simulink model "Autopilotage"  (R2022a)
settings: Solver=VariableStepAuto  StartTime=0.0  StopTime=2  FixedStep=1e-5  MaxStep=1e-4  RelTol=1e-3
undefined symbols (not defined in the file): R0
libraries: spsIGBTDiodeLib x6, spsPWMGenerator2LevelLib x3, spsAsynchronousMachineSIUnitsLib x1, spsDCVoltageSourceLib x1, spsRMSLib x1, spsVoltageMeasurementLib x1, spspowerguiLib x1
settings Model: Creator=kholo  LastModifiedBy=Dell

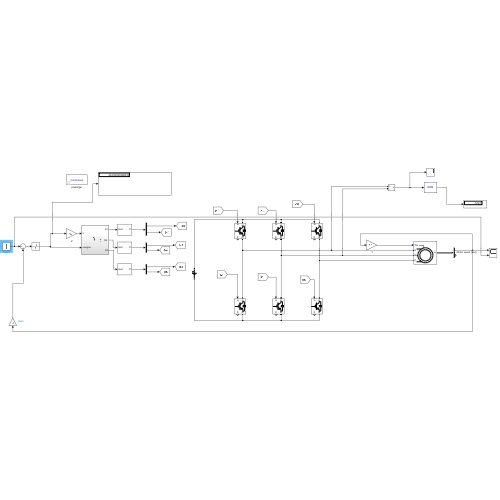
[thumbnail: Simulink's stored preview of the top-level diagram]
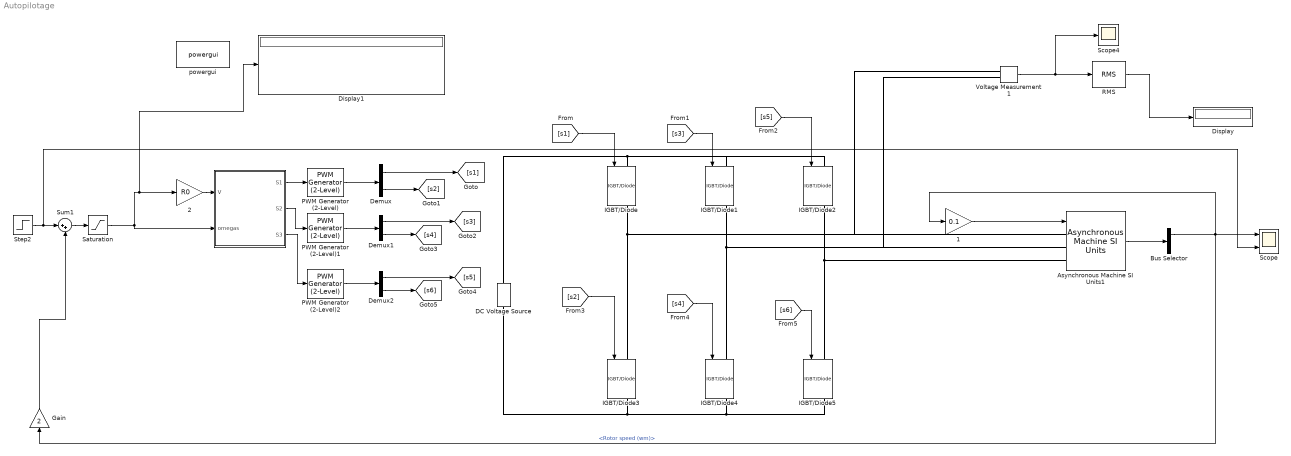
== system Autopilotage ==
  "  " : Subsystem
  " 1" : Gain  Gain=0.1
  " 2" : Gain  Gain=R0
  Asynchronous Machine SI Units1 : spsAsynchronousMachineSIUnitsLib/Asynchronous Machine SI Units  RotorType=Squirrel-cage  PresetModel=No  MechanicalLoad=Torque Tm  ShowDetailedParameters=on  ReferenceFrame=Rotor  Units=SI  MeasurementBus=off  NominalParameters=[1.845e+04 400 50]  VoltageRatio=1  Stator=[0.5968 0.0003495]  Rotor=[0.6258 0.005473]  Cage1=[0.4155 0.002066]  Cage2=[0.4168 0.0003495]  Lm=0.0354  Mechanical=[0.05 0.005879 2]  PolePairs=2  InitialConditions=[0 0 0 0 0 0 0 0]  SimulateSaturation=off  Saturation=[14.03593122, 27.81365428, 53.79336849, 72.68890987, 97.98006896, 148.6815601, 215.7428561, 302.9841135, 428.7778367 ; 230, 322, 414, 460, 506, 552, 598, 644, 690]  LoadFlowParameters=1492000  TsPowergui=0  TsBlock=-1  IterativeModel=Trapezoidal non iterative  IterativeDiscreteModel=Trapezoidal non iterative  Pmec=1.492e+006
      link override Mechanical model/Rotor speed (wm): InitialCondition=SM.wmo*eps
  Bus Selector : BusSelector  OutputSignals=Mechanical.Rotor speed (wm),Mechanical.Electromagnetic torque Te (N*m)
  DC Voltage Source : spsDCVoltageSourceLib/DC Voltage Source  Amplitude=600  Measurements=None
  Demux : Demux  Outputs=2
  Demux1 : Demux  Outputs=2
  Demux2 : Demux  Outputs=2
  Display : Display
  Display1 : Display
  Gain : Gain  Gain=2
  IGBT/Diode{,1..5} (6 alike) : spsIGBTDiodeLib/IGBT//Diode  Ron=1e-3  Rs=1e5  Cs=inf  Measurements=on
  PWM Generator (2-Level) : spsPWMGenerator2LevelLib/PWM Generator (2-Level)  ModulatorType=Single-phase half-bridge (2 pulses)  ModulatorMode=Unsynchronized  Fc=2*60*50  Pc=90  nF=27  MinMax="[ -1  1 ]"  SamplingTechnique=Natural  ModulatingSignals=off  m=0.8  Freq=60  Phase=0  Ts=0  ShowCarrierOutport=off
  PWM Generator (2-Level)1 : spsPWMGenerator2LevelLib/PWM Generator (2-Level)  ModulatorType=Single-phase half-bridge (2 pulses)  ModulatorMode=Unsynchronized  Fc=2*60*50  Pc=90  nF=27  MinMax="[ -1  1 ]"  SamplingTechnique=Natural  ModulatingSignals=off  m=0.8  Freq=60  Phase=0  Ts=0  ShowCarrierOutport=off
  PWM Generator (2-Level)2 : spsPWMGenerator2LevelLib/PWM Generator (2-Level)  ModulatorType=Single-phase half-bridge (2 pulses)  ModulatorMode=Unsynchronized  Fc=2*60*50  Pc=90  nF=27  MinMax="[ -1  1 ]"  SamplingTechnique=Natural  ModulatingSignals=off  m=0.8  Freq=60  Phase=0  Ts=0  ShowCarrierOutport=off
  RMS : spsRMSLib/RMS  TrueRMS=on  Freq=50  RMSInit=120  Ts=0
  Saturation : Saturate  UpperLimit=314  LowerLimit=0
  Scope : Scope  NumInputPorts=2
  Scope4 : Scope
  Step2 : Step  Time=0  Before=15  After=15  SampleTime=0
  Sum1 : Sum  Inputs=|++
  Voltage Measurement1 : spsVoltageMeasurementLib/Voltage Measurement  PhasorSimulation=off  OutputType=Complex  PSBequivalent=0
  powergui : spspowerguiLib/powergui  Priority=1  SimulationMode=Continuous  SampleTime=50e-6  frequency=60  Iterations=50  frequencyindice=50  Pbase=100e6  ErrMax=1e-4  UnitsV=kV  UnitsW=MW  buscounter=0  FunctionMessages=off  echomessages=off  EnableUseOfTLC=off  CurrentSourceSwitches=off  DisableSnubberDevices=off  DisableRonSwitches=off  DisableVfSwitches=off  DisplayEquations=off  AutomaticDiscreteSolvers=off  SolverType=Tustin/Backward Euler (TBE)  Interpol=off  ExternalGateDelay=off  methode=off  Ts=100  x0status=blocks  SPID=on  SwTol=0  HookPort=off  NonlinearTolerance=1e-4  nMaxIteration=100  ContinueOnMaxIteration=off  RestoreLinks=warning  ResistiveCurrentMeasurement=off  Frange=[0:2:500]  Ylog=off  Xlog=on  ShowGrid=off  save=off  variable=ZData  structure=0  ZoomFFT=off  StartTime=0.0  cycles=1  DisplayStyle=1  fundamental=60  FreqAxis=off  MaxFrequency=1000  frequencyindicesteady=1  RmsSteady=1  display=off
  wires:
  Asynchronous Machine SI Units1/1 -> Bus Selector/1
  [s6] -> IGBT/Diode5/1
  [s3] -> IGBT/Diode1/1
  [s5] -> IGBT/Diode2/1
  [s4] -> IGBT/Diode4/1
  [s2] -> IGBT/Diode3/1
  [s1] -> IGBT/Diode/1
  Voltage Measurement1/1 -> Scope4/1, RMS/1
  PWM Generator (2-Level)/1 -> Demux/1
  Demux/1 -> [s1]
  Demux/2 -> [s2]
  PWM Generator (2-Level)1/1 -> Demux1/1
  Demux1/1 -> [s3]
  Demux1/2 -> [s4]
  PWM Generator (2-Level)2/1 -> Demux2/1
  Demux2/1 -> [s5]
  Demux2/2 -> [s6]
  RMS/1 -> Display/1
  "  "/1(S1) -> PWM Generator (2-Level)/1
  "  "/2("S2 ") -> PWM Generator (2-Level)1/1
  "  "/3(S3) -> PWM Generator (2-Level)2/1
  Bus Selector/1 -> Scope/1, " 1"/1, Gain/1  "<Rotor speed (wm)>"
  " 2"/1 -> "  "/1(V)
  " 1"/1 -> Asynchronous Machine SI Units1/1
  Gain/1 -> Sum1/2
  Sum1/1 -> Saturation/1
  Step2/1 -> Scope/2, Sum1/1
  Saturation/1 -> "  "/2(omegas), Display1/1, " 2"/1
  connections:
  IGBT/Diode/LConn1 -- DC Voltage Source/RConn1 -- IGBT/Diode2/LConn1 -- IGBT/Diode1/LConn1
  IGBT/Diode4/LConn1 -- Voltage Measurement1/LConn2 -- Asynchronous Machine SI Units1/LConn2 -- IGBT/Diode1/RConn1
  IGBT/Diode4/RConn1 -- IGBT/Diode5/RConn1 -- DC Voltage Source/LConn1 -- IGBT/Diode3/RConn1
  IGBT/Diode5/LConn1 -- IGBT/Diode2/RConn1 -- Asynchronous Machine SI Units1/LConn3
  IGBT/Diode3/LConn1 -- Voltage Measurement1/LConn1 -- Asynchronous Machine SI Units1/LConn1 -- IGBT/Diode/RConn1

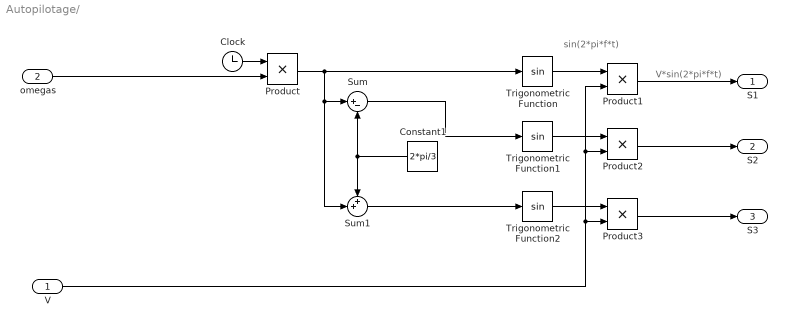
== system Autopilotage/   ==
  note: V*sin(2*pi*f*t)
  note: sin(2*pi*f*t)
  V : Inport
  omegas : Inport  Port=2
  Clock : Clock
  Constant1 : Constant  Value=2*pi/3
  Product{,1..3} (4 alike) : Product
  Sum : Sum  Inputs=|+-
  Sum1 : Sum  Inputs=++|
  Trigonometric Function : Trigonometry
  Trigonometric Function1 : Trigonometry
  Trigonometric Function2 : Trigonometry
  S1 : Outport
  "S2 " : Outport  Port=2
  S3 : Outport  Port=3
  wires:
  Sum1/1 -> Trigonometric Function2/1
  Product1/1 -> S1/1
  omegas/1 -> Product/2
  Trigonometric Function2/1 -> Product3/1
  V/1 -> Product3/2, Product2/2, Product1/2
  Constant1/1 -> Sum/2, Sum1/1
  Trigonometric Function/1 -> Product1/1
  Product3/1 -> S3/1
  Clock/1 -> Product/1
  Sum/1 -> Trigonometric Function1/1
  Trigonometric Function1/1 -> Product2/1
  Product2/1 -> "S2 "/1
  Product/1 -> Sum1/2, Sum/1, Trigonometric Function/1
